simulink model "bwb11"  (Simulink 7.8)
settings: Solver=ode45  StartTime=0.0  StopTime=10.0  RelTol=1e-3
values from neighbouring files (symbols this model uses):
  eagleray = aerosonde_data    [aerosonde_initialize.m]
  euler_0 = [theta_trim; 0; 0]    [aerosonde_initialize.m]
  fuel_0 = 2    [aerosonde_initialize.m]
  Omega_0 = 5000*pi/30    (= 523.598775598)    [aerosonde_initialize.m]
  position_0 = [0; 0; -h_trim]    [aerosonde_initialize.m]
  rates_0 = [0; q_trim ; 0]    [aerosonde_initialize.m]
  velocity_0 = [23; 0; 0]    [aerosonde_initialize.m]
undefined symbols (not defined in the file or in its folder): ke, rAC, tc, z
libraries: aerolibasang x3, aerolibadynsys x3, aerolibbdyn x2, aerolibutil x2, aerolibtransform2 x1, aerolib6dof2 x1, aerolibatmos2 x1
settings Model: Creator=Shihan Tissera  LastModifiedBy=s153429
settings OptimizationCC: InitFltsAndDblsToZero=on
settings DebuggingCC: FcnCallInpInsideContextMsg=Use local settings  StrictBusMsg=Warning

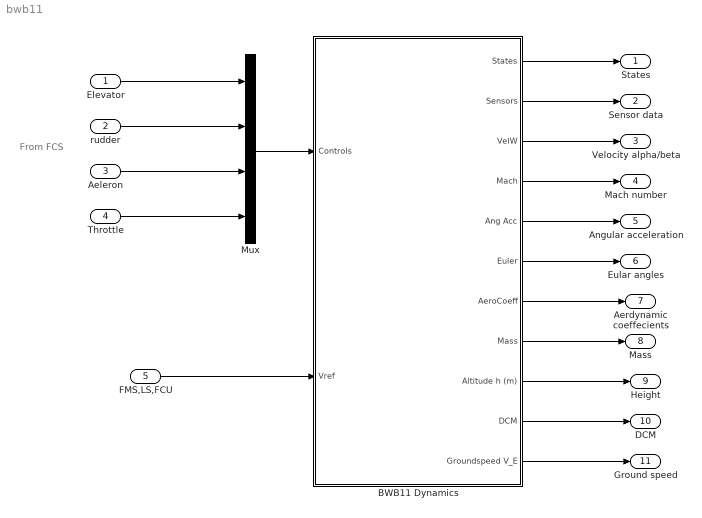
== system bwb11 ==
  note: From FCS
  Elevator : Inport
  rudder : Inport  Port=2
  Aeleron : Inport  Port=3
  Throttle : Inport  Port=4
  FMS,LS,FCU : Inport  Port=5
  BWB11 Dynamics : Subsystem  mask(6-DOF Aerosonde Model){as=eagleray, Velocities0=velocity_0, Rates0=rates_0, Euler0=euler_0, Position0=position_0, Fuel0=fuel_0, Omega0=Omega_0, GndAlt=0}
      mask prompts: as "Aircraft configuration data:"; Velocities0 "Initial velocity in body axes [u,v,w]: (m/s)"; Rates0 "Initial body rotation rates [p,q,r]: (rad/s)"; Euler0 "Initial Euler orientation [roll, pitch, yaw]: (rad)"; Position0 "Initial position in inertial axes [Xe,Ye,Ze]: (m)"; Fuel0 "Initial fuel mass: (Kg)"; Omega0 "Initial engine speed: (rad/s)"; GndAlt "Ground altitude: (m)"
      mask help:
      | Nonlinear 6-DOF Aerosonde  model with equations of motion in
      | body frame.
      |
      | Version 2011a (18 February 2011)
      mask Help:
      | The block implements the 6-DOF nonlinear Aerosonde model. It is an adaptation of the model provided in the AeroSim blockset. Velocities are computed in body frame.
      | <P><B>Inputs:</B>
      | <LI>Controls = the 4x1 vector of aircraft controls [elevator aileron rudder throttle]. Aerodynamic controls are in radians, throttle is from 0 to 1.</LI>
      | <LI>RST = the integrator reset flag (0 or 1, all integrators on rising edge)
      | <LI>V_wind = the 3x1 vector of background wind speed components in navigation frame [North East Down]</LI>
      | <LI>omega_wind = the 3x1 vector of background wind angular rates in navigation frame [North East Down]</LI>
      | </P>
      | <P><B>Outputs:</B>
      | <LI>States = the 14x1 aircraft state vector [Velocities, Angular rates, Euler angles, Position, Fuel mass, Engine speed].</LI>
      | <LI>Sensors = the 15x1 vector of sensor outputs [GPS Position, GPS Groundspeed, Accelerometers, Gyros, Air data].</LI>
      | <LI>VelW = the 3x1 vector of aircraft velocity in wind axes [Airspeed, sideslip, angle of attack]</LI>
      | <LI>Mach = the Mach number</LI>
      | <LI>Ang Acc = the 3x1 vector of angular accelerations
      | <LI>Euler = the 3x1 vector of Euler angles (roll, pitch, yaw)</LI>
      | <LI>AeroCoeff = the 6x1 vector of aerodynamic coefficients [CD CY CL Cl Cm Cn]</LI>
      | <LI>Mass = the current aircraft mass</LI>
      | <LI>h = the aircraft altitude</LI>
      | </P>
      | <P><B>Parameters:</B>
      | <LI>Aircraft configuration data = structured varaible with aircraft data<BR>
      | obtain by  ``aerosonde=aerosonde_initialize'' for example</LI>
      | <LI>Initial velocities = the 3x1 vector of initial aircraft velocities in body axes [u v w]</LI>
      | <LI>Initial angular rates = the 3x1 vector of initial angular rates [p q r]</LI>
      | <LI>Initial attitude = the 3x1 vector of initial Euler angles [phi theta psi]</LI>
      | <LI>Initial position = the 3x1 vector of initial aircraft location [Lat Lon Alt]</LI>
      | <LI>Initial fuel mass = the initial quantity of fuel on-board the aircraft</LI>
      | <LI>Initial engine speed = the initial engine rotation speed</LI>
      | <LI>Ground altitude = the ground altitude at aircraft location</LI>
      | </P>
      | <P>
      | <I>Version 2010b (26 May 2010)</I>
      | </P>
  Mux : Mux
  States : Outport
  Sensor data : Outport  Port=2
  Velocity alpha/beta : Outport  Port=3
  Mach number : Outport  Port=4
  Angular acceleration : Outport  Port=5
  Eular angles : Outport  Port=6
  Aerdynamic coeffecients : Outport  Port=7
  Mass : Outport  Port=8
  Height : Outport  Port=9
  DCM : Outport  Port=10
  Ground speed : Outport  Port=11
  wires:
  BWB11 Dynamics/1(States) -> States/1
  BWB11 Dynamics/2(Sensors) -> Sensor data/1
  BWB11 Dynamics/3(VelW) -> Velocity alpha/beta/1
  BWB11 Dynamics/4(Mach) -> Mach number/1
  BWB11 Dynamics/5(Ang Acc) -> Angular acceleration/1
  BWB11 Dynamics/6(Euler) -> Eular angles/1
  BWB11 Dynamics/7(AeroCoeff) -> Aerdynamic coeffecients/1
  BWB11 Dynamics/8(Mass) -> Mass/1
  BWB11 Dynamics/9("Altitude h (m) ") -> Height/1
  BWB11 Dynamics/10(DCM) -> DCM/1
  BWB11 Dynamics/11(Groundspeed V_E) -> Ground speed/1
  Mux/1 -> BWB11 Dynamics/1(Controls)
  Elevator/1 -> Mux/1
  rudder/1 -> Mux/2
  Aeleron/1 -> Mux/3
  Throttle/1 -> Mux/4
  FMS,LS,FCU/1 -> BWB11 Dynamics/2(Vref)

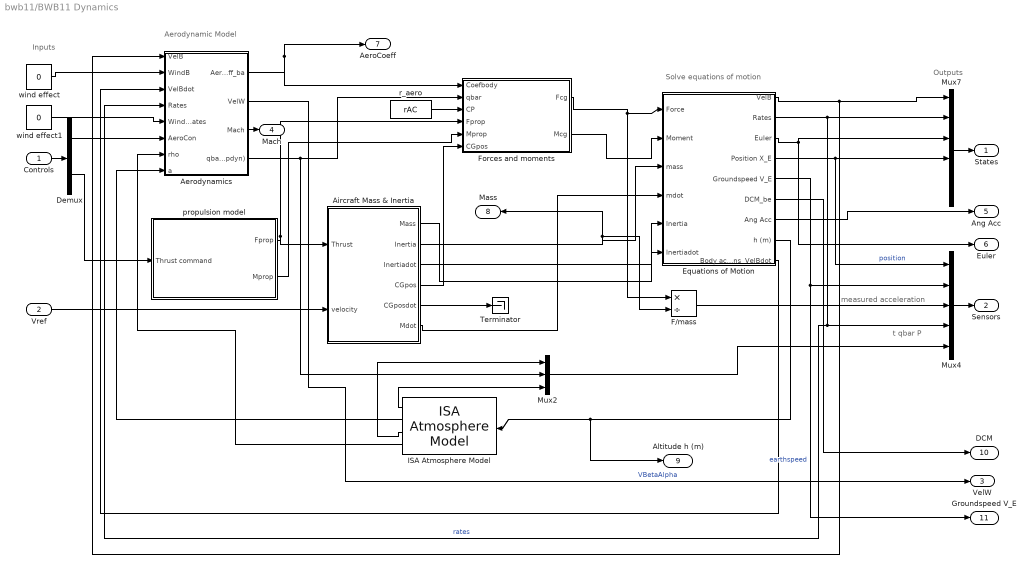
== system bwb11/BWB11 Dynamics ==
  note: t qbar P
  note: measured acceleration
  note: Aerodynamic Model
  note: Outputs
  note: Inputs
  note: Solve equations of motion
  Controls : Inport
  Vref : Inport  Port=2
  Aerodynamics : Subsystem
  Aircraft Mass & Inertia : Subsystem
  Demux : Demux  Outputs=[4,3]
  Equations of Motion : Subsystem
  F/mass : Product  Inputs=*/  RndMeth=Zero
  Forces and moments : Subsystem
  ISA Atmosphere Model : aerolibatmos2/ISA Atmosphere Model  custom=off  g=9.80665  gamma=1.4  R=287.0531  L=0.0065  h_trop=11000  h_strat=20000  rho0=1.225  P0=101325  T0=288.15
  Mux2 : Mux  Inputs=3
  Mux4 : Mux  Inputs=5
  Mux7 : Mux  Inputs=6
  Terminator : Terminator
  propulsion model : Subsystem
  r_aero : Constant  Value=rAC
  wind effect : Constant  Value=0
  wind effect1 : Constant  Value=0
  States : Outport
  Sensors : Outport  Port=2
  VelW : Outport  Port=3
  Mach : Outport  Port=4
  Ang Acc : Outport  Port=5
  Euler : Outport  Port=6
  AeroCoeff : Outport  Port=7
  Mass : Outport  Port=8
  "Altitude h (m) " : Outport  Port=9
  DCM : Outport  Port=10
  Groundspeed V_E : Outport  Port=11
  wires:
  wind effect/1 -> Aerodynamics/2(WindB)
  wind effect1/1 -> Aerodynamics/5(WindRates)
  Equations of Motion/9(Body accns  VelBdot) -> Aerodynamics/3(VelBdot)
  F/mass/1 -> Mux4/3
  Aircraft Mass & Inertia/2(Inertia) -> Equations of Motion/5(Inertia)
  Forces and moments/1(Fcg) -> F/mass/1, Equations of Motion/1(Force)
  r_aero/1 -> Forces and moments/3(CP)
  Equations of Motion/8(h (m)) -> "Altitude h (m) "/1, ISA Atmosphere Model/1
  ISA Atmosphere Model/4 -> Aerodynamics/7(rho)
  ISA Atmosphere Model/3 -> Mux2/1
  ISA Atmosphere Model/2 -> Aerodynamics/8("a ")
  ISA Atmosphere Model/1 -> Mux2/3
  Aerodynamics/1(AeroCoeff_ba) -> AeroCoeff/1, Forces and moments/1(Coefbody)
  Aerodynamics/3(Mach) -> Mach/1
  Demux/1 -> Aerodynamics/6(AeroCon)
  Equations of Motion/4(Position X_E) -> Mux4/1, Mux7/4  "position"
  Equations of Motion/2(Rates) -> Mux7/2, Mux4/4, Aerodynamics/4(Rates)  "rates"
  Equations of Motion/1(VelB) -> Aerodynamics/1(VelB), Mux7/1
  Demux/2 -> propulsion model/1(Thrust command)
  Mux7/1 -> States/1
  Mux4/1 -> Sensors/1
  Controls/1 -> Demux/1
  Equations of Motion/5(Groundspeed V_E) -> Groundspeed V_E/1, Mux4/2  "earthspeed"
  Aircraft Mass & Inertia/1(Mass) -> F/mass/2, Equations of Motion/3(mass), Mass/1
  Forces and moments/2(Mcg) -> Equations of Motion/2(Moment)
  propulsion model/1(Fprop) -> Forces and moments/4(Fprop), Aircraft Mass & Inertia/1(Thrust)
  propulsion model/2(Mprop) -> Forces and moments/5(Mprop)
  Equations of Motion/6(DCM_be) -> DCM/1
  Aerodynamics/4(qbar (pdyn)) -> Mux2/2, Forces and moments/2(qbar)
  Mux2/1 -> Mux4/5
  Aerodynamics/2(VelW) -> VelW/1  "VBetaAlpha"
  Equations of Motion/7(Ang Acc) -> Ang Acc/1
  Equations of Motion/3(Euler) -> Mux7/3, Euler/1
  Aircraft Mass & Inertia/4(CGpos) -> Forces and moments/6(CGpos)
  Aircraft Mass & Inertia/6(Mdot) -> Equations of Motion/4(mdot)
  Aircraft Mass & Inertia/5(CGposdot) -> Terminator/1
  Aircraft Mass & Inertia/3(Inertiadot) -> Equations of Motion/6(Inertiadot)
  Vref/1 -> Aircraft Mass & Inertia/2(velocity)

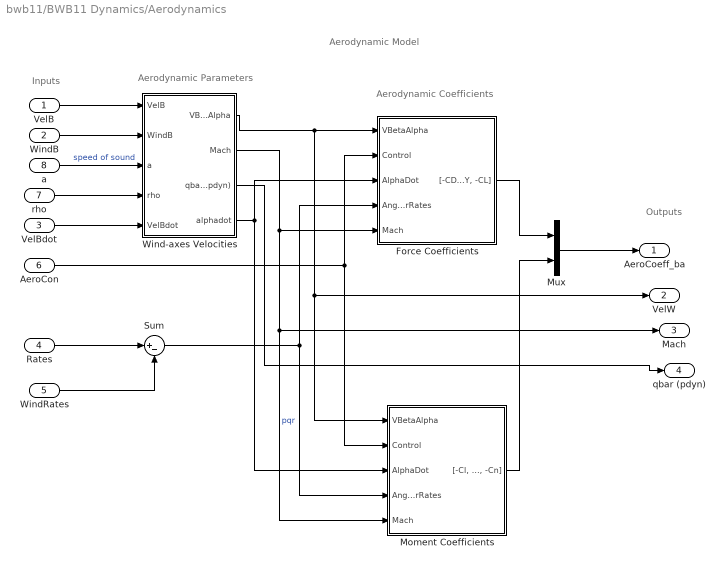
== system bwb11/BWB11 Dynamics/Aerodynamics ==
  note: Aerodynamic Model
  note: Aerodynamic Coefficients
  note: Aerodynamic Parameters
  note: Outputs
  note: Inputs
  VelB : Inport  PortDimensions=[3 1]
  WindB : Inport  Port=2  PortDimensions=[3 1]
  VelBdot : Inport  Port=3
  Rates : Inport  Port=4  PortDimensions=[3 1]
  WindRates : Inport  Port=5  PortDimensions=[3 1]
  AeroCon : Inport  Port=6  PortDimensions=[4 1]
  rho : Inport  Port=7  PortDimensions=1
  "a " : Inport  Port=8  PortDimensions=1
  Force Coefficients : Subsystem
  Moment Coefficients : Subsystem
  Mux : Mux  Inputs=2
  Sum : Sum  Inputs=|+-  SaturateOnIntegerOverflow=on  InputSameDT=on  OutDataTypeStr=Inherit: Same as first input
  Wind-axes Velocities : Subsystem
  AeroCoeff_ba : Outport
  VelW : Outport  Port=2
  Mach : Outport  Port=3
  qbar (pdyn) : Outport  Port=4
  wires:
  VelBdot/1 -> Wind-axes Velocities/5(VelBdot)
  Wind-axes Velocities/4(alphadot) -> Force Coefficients/3(AlphaDot), Moment Coefficients/3(AlphaDot)
  WindB/1 -> Wind-axes Velocities/2(WindB)
  Mux/1 -> AeroCoeff_ba/1
  Moment Coefficients/1("[-Cl, Cm, -Cn]") -> Mux/2
  Force Coefficients/1("[-CD, CY, -CL]") -> Mux/1
  rho/1 -> Wind-axes Velocities/4(rho)
  VelB/1 -> Wind-axes Velocities/1(VelB)
  "a "/1 -> Wind-axes Velocities/3(a)  "speed of sound"
  Wind-axes Velocities/1(VBetaAlpha) -> Moment Coefficients/1(VBetaAlpha), VelW/1, Force Coefficients/1(VBetaAlpha)
  AeroCon/1 -> Moment Coefficients/2(Control), Force Coefficients/2(Control)
  Wind-axes Velocities/2(Mach) -> Moment Coefficients/5(Mach), Force Coefficients/5(Mach), Mach/1
  Wind-axes Velocities/3(qbar (pdyn)) -> qbar (pdyn)/1
  Rates/1 -> Sum/1
  Sum/1 -> Moment Coefficients/4(AngularRates), Force Coefficients/4(AngularRates)  "pqr"
  WindRates/1 -> Sum/2

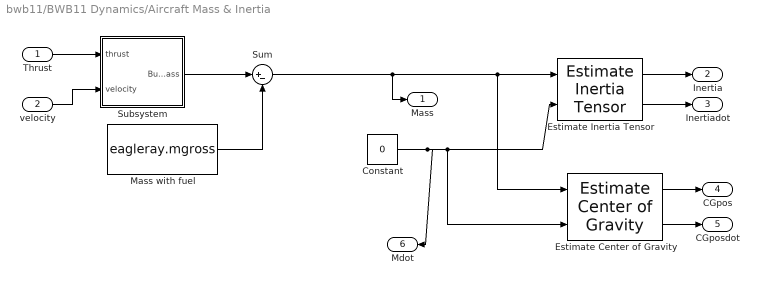
== system bwb11/BWB11 Dynamics/Aircraft Mass & Inertia ==
  Thrust : Inport
  velocity : Inport  Port=2
  Constant : Constant  Value=0
  Estimate Center of Gravity : aerolibbdyn/Estimate Center of Gravity  fmass=eagleray.mgross  emass=eagleray.mempty  fcg=eagleray.CGgross  ecg=eagleray.CGempty
  Estimate Inertia Tensor : aerolibbdyn/Estimate Inertia Tensor  fmass=eagleray.mgross  emass=eagleray.mempty  fI=eagleray.Jgross  eI=eagleray.Jempty
  Mass with fuel : Constant  Value=eagleray.mgross
  Subsystem : Subsystem
  Sum : Sum  Inputs=|+-  SaturateOnIntegerOverflow=on  InputSameDT=on  OutDataTypeStr=Inherit: Same as first input
  Mass : Outport
  Inertia : Outport  Port=2
  Inertiadot : Outport  Port=3
  CGpos : Outport  Port=4
  CGposdot : Outport  Port=5
  Mdot : Outport  Port=6
  wires:
  Estimate Center of Gravity/2 -> CGposdot/1
  Estimate Center of Gravity/1 -> CGpos/1
  Estimate Inertia Tensor/2 -> Inertiadot/1
  Estimate Inertia Tensor/1 -> Inertia/1
  Sum/1 -> Estimate Center of Gravity/1, Estimate Inertia Tensor/1, Mass/1
  Mass with fuel/1 -> Sum/2
  Subsystem/1(Burned fuel mass) -> Sum/1
  Constant/1 -> Estimate Inertia Tensor/2, Estimate Center of Gravity/2, Mdot/1
  Thrust/1 -> Subsystem/1(thrust)
  velocity/1 -> Subsystem/2(velocity)

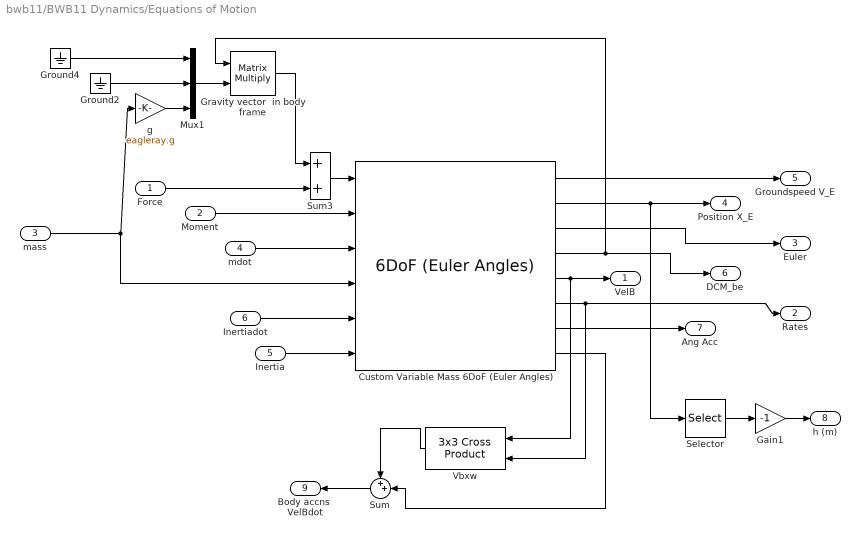
== system bwb11/BWB11 Dynamics/Equations of Motion ==
  Force : Inport  PortDimensions=3
  Moment : Inport  Port=2  PortDimensions=3
  mass : Inport  Port=3  PortDimensions=1
  mdot : Inport  Port=4  PortDimensions=1
  Inertia : Inport  Port=5  PortDimensions=[3,3]
  Inertiadot : Inport  Port=6  PortDimensions=[3,3]
  Custom Variable Mass 6DoF (Euler Angles) : aerolib6dof2/6DoF (Euler Angles)  units=Metric (MKS)  mtype=Custom Variable  rep=Euler Angles  xme_0=Position0  Vm_0=Velocities0  eul_0=Euler0  pm_0=Rates0  mass_0=1.0  mass_e=0  mass_f=0  inertia=eye(3)  inertia_e=eye(3)  inertia_f=eye(3)  k_quat=1.0
  Gain1 : Gain  Gain=-1
  "Gravity vector  in body frame " : Product  Multiplication=Matrix(*)  SaturateOnIntegerOverflow=on  InputSameDT=on  OutDataTypeStr=Inherit: Same as first input
  Ground2 : Ground
  Ground4 : Ground
  Mux1 : Mux  Inputs=3
  Selector : Selector  InputPortWidth=3  IndexOptions=Index vector (dialog)  Indices=3  OutputSizes=1
  Sum : Sum  Inputs=++|  SaturateOnIntegerOverflow=on
  Sum3 : Sum  SaturateOnIntegerOverflow=on  InputSameDT=on  OutDataTypeStr=Inherit: Same as first input
  Vbxw : aerolibutil/3x3 Cross Product
  g : Gain  Gain=eagleray.g
  VelB : Outport
  Rates : Outport  Port=2
  Euler : Outport  Port=3
  Position X_E : Outport  Port=4
  Groundspeed V_E : Outport  Port=5
  DCM_be : Outport  Port=6
  Ang Acc : Outport  Port=7
  h (m) : Outport  Port=8
  Body accns  VelBdot : Outport  Port=9
  wires:
  Vbxw/1 -> Sum/1
  Sum/1 -> Body accns  VelBdot/1
  Custom Variable Mass 6DoF (Euler Angles)/8 -> Sum/2
  Custom Variable Mass 6DoF (Euler Angles)/7 -> Ang Acc/1
  Custom Variable Mass 6DoF (Euler Angles)/6 -> Vbxw/2, Rates/1
  Inertia/1 -> Custom Variable Mass 6DoF (Euler Angles)/6
  mdot/1 -> Custom Variable Mass 6DoF (Euler Angles)/3
  Gain1/1 -> h (m)/1
  Selector/1 -> Gain1/1
  Sum3/1 -> Custom Variable Mass 6DoF (Euler Angles)/1
  g/1 -> Mux1/3
  "Gravity vector  in body frame "/1 -> Sum3/1
  Custom Variable Mass 6DoF (Euler Angles)/3 -> Euler/1
  Custom Variable Mass 6DoF (Euler Angles)/2 -> Selector/1, Position X_E/1
  Custom Variable Mass 6DoF (Euler Angles)/1 -> Groundspeed V_E/1
  Custom Variable Mass 6DoF (Euler Angles)/5 -> Vbxw/1, VelB/1
  Ground4/1 -> Mux1/1
  Ground2/1 -> Mux1/2
  mass/1 -> Custom Variable Mass 6DoF (Euler Angles)/4, g/1
  Custom Variable Mass 6DoF (Euler Angles)/4 -> DCM_be/1, "Gravity vector  in body frame "/1
  Mux1/1 -> "Gravity vector  in body frame "/2
  Force/1 -> Sum3/2
  Moment/1 -> Custom Variable Mass 6DoF (Euler Angles)/2
  Inertiadot/1 -> Custom Variable Mass 6DoF (Euler Angles)/5

== system bwb11/BWB11 Dynamics/Forces and moments ==
  Coefbody : Inport
  qbar : Inport  Port=2
  CP : Inport  Port=3
  Fprop : Inport  Port=4
  Mprop : Inport  Port=5
  CGpos : Inport  Port=6
  Aerodynamic Forces and Moments : Subsystem  AncestorBlock=aerolibadyn/Aerodynamic Forces and Moments  mask(Aerodynamic Forces and Moments){inputAxes=Body, outputForceAxes=Body, outputMomentAxes=Body, S=eagleray.S, b=eagleray.b, cbar=eagleray.MAC}
      mask prompts: inputAxes "Input axes:"; outputForceAxes "Force axes:"; outputMomentAxes "Moment axes:"; S "Reference area:"; b "Reference span:"; cbar "Reference length:"
      mask help: Compute the aerodynamic forces and moments applied at the center of gravity using the aerodynamic coefficients, dynamic pressure, center of gravity and center of pressure.
      mask init:
      | ports=aeroicon('aeroblkadyn','icon');
      mask Help: eval('asbhelp');
      mask StyleString: popup(Body|Stability|Wind),popup(Body|Stability|Wind),popup(Body|Stability|Wind),edit,edit,edit
      mask Display:
      | port_label(ports(1).type,ports(1).port,ports(1).txt,'texmode','on');
      | port_label(ports(2).type,ports(2).port,ports(2).txt,'texmode','on');
      | port_label(ports(3).type,ports(3).port,ports(3).txt,'texmode','on');
      | port_label(ports(4).type,ports(4).port,ports(4).txt,'texmode','on');
      | port_label(ports(5).type,ports(5).port,ports(5).txt,'texmode','on');
      | port_label(ports(6).type,ports(6).port,ports(6).txt,'texmode','on');
      | port_label(ports(7).type,ports(7).port,ports(7).txt,'texmode','on');
  Total Moment : Subsystem
  Fcg : Outport
  Mcg : Outport  Port=2
  wires:
  Aerodynamic Forces and Moments/2(Moments) -> Total Moment/2(Maero)
  Aerodynamic Forces and Moments/1(Forces) -> Total Moment/1(Faero)
  CGpos/1 -> Total Moment/5(CGpos), Aerodynamic Forces and Moments/3(CG)
  Coefbody/1 -> Aerodynamic Forces and Moments/1(Coefficients)
  qbar/1 -> Aerodynamic Forces and Moments/2(qbar)
  CP/1 -> Aerodynamic Forces and Moments/4(CP)
  Fprop/1 -> Total Moment/3(Fprop)
  Mprop/1 -> Total Moment/4(Mprop)
  Total Moment/2(Mcg) -> Mcg/1
  Total Moment/1(Fcg) -> Fcg/1

== system bwb11/BWB11 Dynamics/propulsion model ==
  Thrust command : Inport
  CGtoFdistance : Constant  Value=z
  Engine model : TransferFcn  Numerator=[ke]  Denominator=[tc 1]
  Product : Product  RndMeth=Zero
  Fprop : Outport
  Mprop : Outport  Port=2
  wires:
  CGtoFdistance/1 -> Product/2
  Engine model/1 -> Product/1, Fprop/1
  Product/1 -> Mprop/1
  Thrust command/1 -> Engine model/1

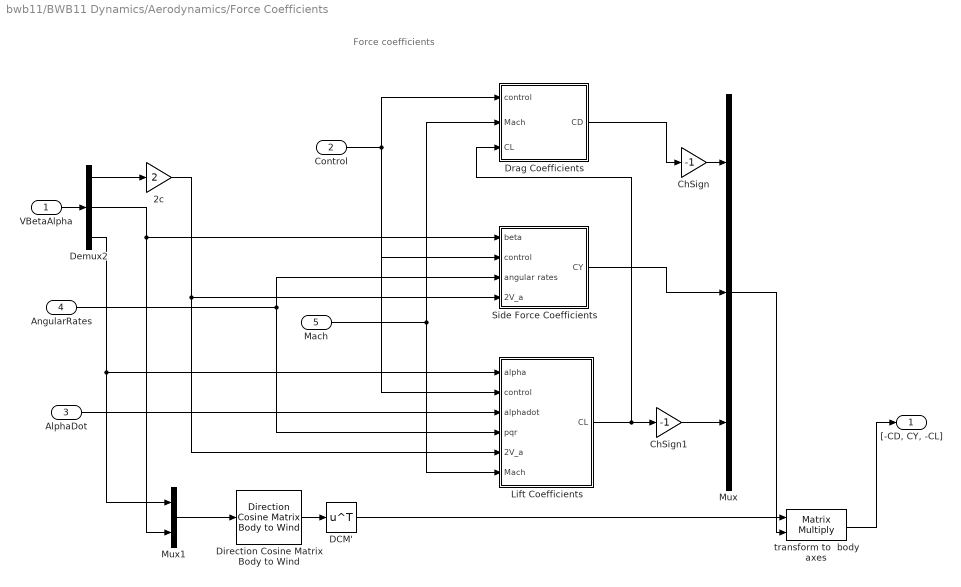
== system bwb11/BWB11 Dynamics/Aerodynamics/Force Coefficients ==
  note: Force coefficients
  VBetaAlpha : Inport  PortDimensions=[3 1]
  Control : Inport  Port=2  PortDimensions=[4 1]
  AlphaDot : Inport  Port=3
  AngularRates : Inport  Port=4  PortDimensions=[3 1]
  Mach : Inport  Port=5  PortDimensions=1
  2c : Gain  Gain=2  SaturateOnIntegerOverflow=on  OutDataTypeStr=Inherit: Same as input  ParamDataTypeStr=Inherit: Same as input
  ChSign : Gain  Gain=-1  SaturateOnIntegerOverflow=on  OutDataTypeStr=Inherit: Same as input  ParamDataTypeStr=Inherit: Same as input
  ChSign1 : Gain  Gain=-1  SaturateOnIntegerOverflow=on  OutDataTypeStr=Inherit: Same as input  ParamDataTypeStr=Inherit: Same as input
  DCM' : Math  Operator=transpose  SaturateOnIntegerOverflow=on
  Demux2 : Demux  Outputs=3
  Direction Cosine Matrix Body to Wind : aerolibtransform2/Direction Cosine Matrix Body to Wind
  Drag Coefficients : Subsystem
  Lift Coefficients : Subsystem
  Mux : Mux  Inputs=3
  Mux1 : Mux  Inputs=2
  Side Force Coefficients : Subsystem
  transform to  body axes : Product  Inputs=**  Multiplication=Matrix(*)  SaturateOnIntegerOverflow=on  InputSameDT=on  OutDataTypeStr=Inherit: Same as first input
  "[-CD, CY, -CL]" : Outport
  wires:
  Mux1/1 -> Direction Cosine Matrix Body to Wind/1
  DCM'/1 -> transform to  body axes/1
  Mux/1 -> transform to  body axes/2
  Direction Cosine Matrix Body to Wind/1 -> DCM'/1
  transform to  body axes/1 -> "[-CD, CY, -CL]"/1
  Demux2/2 -> Mux1/2, Side Force Coefficients/1(beta)
  Demux2/1 -> 2c/1
  VBetaAlpha/1 -> Demux2/1
  ChSign1/1 -> Mux/3
  ChSign/1 -> Mux/1
  Side Force Coefficients/1(CY) -> Mux/2
  Drag Coefficients/1(CD) -> ChSign/1
  Lift Coefficients/1(CL) -> Drag Coefficients/3(CL), ChSign1/1
  Mach/1 -> Drag Coefficients/2(Mach), Lift Coefficients/6(Mach)
  AngularRates/1 -> Side Force Coefficients/3(angular rates), Lift Coefficients/4(pqr)
  AlphaDot/1 -> Lift Coefficients/3(alphadot)
  Control/1 -> Lift Coefficients/2(control), Side Force Coefficients/2(control), Drag Coefficients/1(control)
  Demux2/3 -> Lift Coefficients/1(alpha), Mux1/1
  2c/1 -> Side Force Coefficients/4(2V_a), Lift Coefficients/5(2V_a)

== system bwb11/BWB11 Dynamics/Aerodynamics/Moment Coefficients ==
  note: Moment coefficients
  VBetaAlpha : Inport  PortDimensions=[3 1]
  Control : Inport  Port=2  PortDimensions=[4 1]
  AlphaDot : Inport  Port=3
  AngularRates : Inport  Port=4  PortDimensions=[3 1]
  Mach : Inport  Port=5  PortDimensions=1
  2c : Gain  Gain=2  SaturateOnIntegerOverflow=on  OutDataTypeStr=Inherit: Same as input  ParamDataTypeStr=Inherit: Same as input
  Demux1 : Demux  Outputs=3
  Mux : Mux  Inputs=3
  Pitch Moment Coefficients : Subsystem
  Roll Moment Coefficients : Subsystem
  Yaw Moment Coefficients : Subsystem
  "[-Cl, Cm, -Cn]" : Outport
  wires:
  Demux1/2 -> Yaw Moment Coefficients/1(beta), Roll Moment Coefficients/1(beta)
  Demux1/3 -> Pitch Moment Coefficients/1(alpha)
  Mach/1 -> Pitch Moment Coefficients/6(Mach)
  Yaw Moment Coefficients/1(Cn) -> Mux/3
  VBetaAlpha/1 -> Demux1/1
  2c/1 -> Pitch Moment Coefficients/5(2V_a), Yaw Moment Coefficients/4(2V_a), Roll Moment Coefficients/4(2V)
  Demux1/1 -> 2c/1
  Control/1 -> Roll Moment Coefficients/2(control), Yaw Moment Coefficients/2(control), Pitch Moment Coefficients/2(control)
  AlphaDot/1 -> Pitch Moment Coefficients/3(alphadot)
  AngularRates/1 -> Roll Moment Coefficients/3(angular rates), Yaw Moment Coefficients/3(angular rates), Pitch Moment Coefficients/4(pqr)
  Mux/1 -> "[-Cl, Cm, -Cn]"/1
  Pitch Moment Coefficients/1(Cm) -> Mux/2
  Roll Moment Coefficients/1(Cl) -> Mux/1

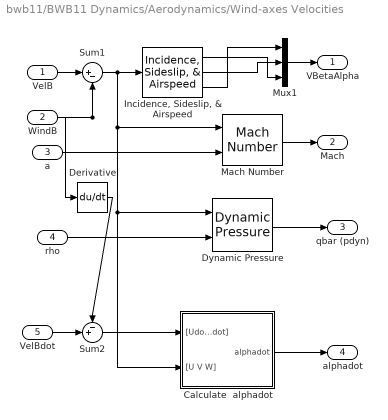
== system bwb11/BWB11 Dynamics/Aerodynamics/Wind-axes Velocities ==
  VelB : Inport
  WindB : Inport  Port=2
  a : Inport  Port=3
  rho : Inport  Port=4
  VelBdot : Inport  Port=5
  Calculate  alphadot : Subsystem
  Derivative : Derivative
  Dynamic Pressure : aerolibasang/Dynamic Pressure
  "Incidence, Sideslip, & Airspeed" : aerolibasang/Incidence, Sideslip, & Airspeed
  Mach Number : aerolibasang/Mach Number
  Mux1 : Mux  Inputs=3
  Sum1 : Sum  Inputs=|+-  SaturateOnIntegerOverflow=on  InputSameDT=on  OutDataTypeStr=Inherit: Same as first input
  Sum2 : Sum  Inputs=-+|  SaturateOnIntegerOverflow=on  InputSameDT=on  OutDataTypeStr=Inherit: Same as first input
  VBetaAlpha : Outport
  Mach : Outport  Port=2
  qbar (pdyn) : Outport  Port=3
  alphadot : Outport  Port=4
  wires:
  Derivative/1 -> Sum2/1
  Sum2/1 -> Calculate  alphadot/1("[Udot Vdot Wdot]")
  VelBdot/1 -> Sum2/2
  Calculate  alphadot/1(alphadot) -> alphadot/1
  "Incidence, Sideslip, & Airspeed"/2 -> Mux1/2
  "Incidence, Sideslip, & Airspeed"/1 -> Mux1/3
  Dynamic Pressure/1 -> qbar (pdyn)/1
  rho/1 -> Dynamic Pressure/2
  a/1 -> Mach Number/2
  Mach Number/1 -> Mach/1
  WindB/1 -> Derivative/1, Sum1/2
  VelB/1 -> Sum1/1
  Mux1/1 -> VBetaAlpha/1
  "Incidence, Sideslip, & Airspeed"/3 -> Mux1/1
  Sum1/1 -> Calculate  alphadot/2("[U V W]"), Dynamic Pressure/1, Mach Number/1, "Incidence, Sideslip, & Airspeed"/1

== system bwb11/BWB11 Dynamics/Aircraft Mass & Inertia/Subsystem ==
  thrust : Inport
  velocity : Inport  Port=2
  Divide : Product  Inputs=*/
  Integrator : Integrator
  Product : Product  RndMeth=Zero
  Product1 : Product  RndMeth=Zero
  calerific value : Constant  Value=eagleray.cali
  "efficency " : Constant  Value=eagleray.Efi
  Burned fuel mass : Outport
  wires:
  thrust/1 -> Product/1
  velocity/1 -> Product/2
  Product/1 -> Integrator/1
  Integrator/1 -> Product1/1
  Divide/1 -> Product1/2
  Product1/1 -> Burned fuel mass/1
  "efficency "/1 -> Divide/1
  calerific value/1 -> Divide/2

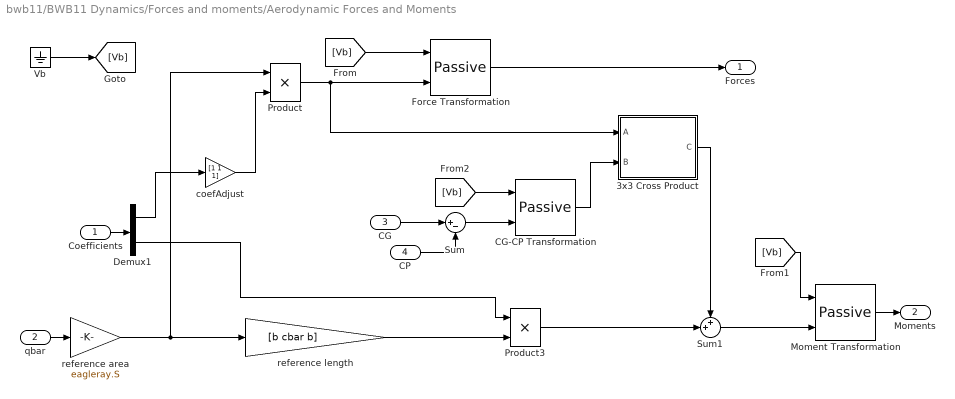
== system bwb11/BWB11 Dynamics/Forces and moments/Aerodynamic Forces and Moments ==
  Coefficients : Inport
  qbar : Inport  Port=2
  CG : Inport  Port=3
  CP : Inport  Port=4
  3x3 Cross Product : Subsystem  AncestorBlock=aerolibutil/3x3 Cross Product  mask(CrossProduct){}
      mask help: Calculate the cross product of two 3-by-1 vectors.
      mask init:
      | aeroicon('aeroblk');
      mask Help: eval('asbhelp(''threebythree_cross_product'')');
      mask Display:
      | text(.5,.5,'Cross\nProduct\nC = AxB', ...
      | 	'HorizontalAlignment','Center',...
      | 	'VerticalAlignment','middle')
  CG-CP Transformation : aerolibadynsys/Passive  SystemSampleTime=-1
  Demux1 : Demux  Outputs=[3,3]
  Force Transformation : aerolibadynsys/Passive  SystemSampleTime=-1
  Moment Transformation : aerolibadynsys/Passive  SystemSampleTime=-1
  Product : Product  SaturateOnIntegerOverflow=on  InputSameDT=on  OutDataTypeStr=Inherit: Same as first input
  Product3 : Product  SaturateOnIntegerOverflow=on  InputSameDT=on  OutDataTypeStr=Inherit: Same as first input
  Sum : Sum  Inputs=|+-  SaturateOnIntegerOverflow=on
  Sum1 : Sum  Inputs=++|  SaturateOnIntegerOverflow=on  InputSameDT=on  OutDataTypeStr=Inherit: Same as first input
  Vb : Ground
  coefAdjust : Gain  Gain="[1  1  1]"
  reference area : Gain  Gain=eagleray.S  SaturateOnIntegerOverflow=on  OutDataTypeStr=Inherit: Same as input  ParamDataTypeStr=Inherit: Same as input
  reference length : Gain  Gain=[b cbar b]  SaturateOnIntegerOverflow=on  OutDataTypeStr=Inherit: Same as input  ParamDataTypeStr=Inherit: Same as input
  Forces : Outport
  Moments : Outport  Port=2
  wires:
  3x3 Cross Product/1(C) -> Sum1/1
  reference length/1 -> Product3/2
  Coefficients/1 -> Demux1/1
  Demux1/2 -> Product3/1
  qbar/1 -> reference area/1
  reference area/1 -> reference length/1, Product/1
  Product3/1 -> Sum1/2
  Demux1/1 -> coefAdjust/1
  Product/1 -> Force Transformation/2, 3x3 Cross Product/1(A)
  Force Transformation/1 -> Forces/1
  Vb/1 -> [Vb]
  [Vb] -> Force Transformation/1
  Sum1/1 -> Moment Transformation/2
  Moment Transformation/1 -> Moments/1
  [Vb] -> Moment Transformation/1
  coefAdjust/1 -> Product/2
  CG/1 -> Sum/1
  CP/1 -> Sum/2
  Sum/1 -> CG-CP Transformation/2
  CG-CP Transformation/1 -> 3x3 Cross Product/2(B)
  [Vb] -> CG-CP Transformation/1

== system bwb11/BWB11 Dynamics/Forces and moments/Total Moment ==
  note: Sum forces and moments
  note: Total moments at CG location
  Faero : Inport  PortDimensions=3
  Maero : Inport  Port=2  PortDimensions=3
  Fprop : Inport  Port=3  PortDimensions=3
  Mprop : Inport  Port=4  PortDimensions=3
  CGpos : Inport  Port=5  PortDimensions=3
  Moments about CG  due to Propulsion   Forces : Subsystem  AncestorBlock="aerolibbdyn/Moments about CG  due to Forces"  mask(Moments About CG Due To Forces){}
      mask help: Compute moments about center of gravity due to forces which are applied at point CP not the center of gravity.
      mask init:
      | [xpw ypw xp yp x y]=aeroimage('momcg');
      mask Help: web(asbhelp);
      mask Display:
      | port_label('input',1,'F','texmode','on');
      | port_label('input',2,'CG','texmode','on');
      | port_label('input',3,'CP','texmode','on');
      | port_label('output',1,'M','texmode','on');
      | patch(xp,yp);
      | patch(xpw,ypw,[1 1 1]);
      | plot(x,y);
  Sum1 : Sum  Inputs=+++  SaturateOnIntegerOverflow=on  InputSameDT=on  OutDataTypeStr=Inherit: Same as first input
  Total forces  (excluding g) : Sum  SaturateOnIntegerOverflow=on  InputSameDT=on  OutDataTypeStr=Inherit: Same as first input
  Fcg : Outport
  Mcg : Outport  Port=2
  wires:
  Maero/1 -> Sum1/2
  Moments about CG  due to Propulsion   Forces/1(Moments) -> Sum1/1
  Total forces  (excluding g)/1 -> Fcg/1
  Faero/1 -> Total forces  (excluding g)/1
  Fprop/1 -> Total forces  (excluding g)/2, Moments about CG  due to Propulsion   Forces/1(Forces)
  Mprop/1 -> Sum1/3
  Sum1/1 -> Mcg/1
  CGpos/1 -> Moments about CG  due to Propulsion   Forces/2(CG)

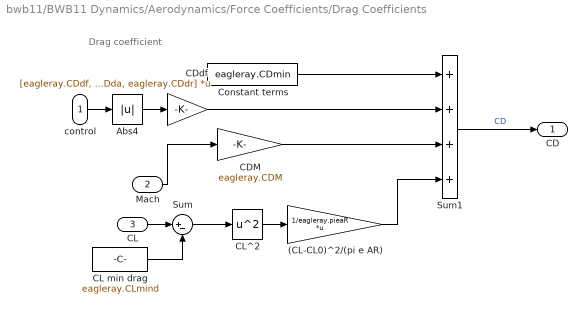
== system bwb11/BWB11 Dynamics/Aerodynamics/Force Coefficients/Drag Coefficients ==
  note: Drag coefficient
  control : Inport
  Mach : Inport  Port=2
  CL : Inport  Port=3  PortDimensions=1
  (CL-CL0)^2/(pi e AR) : Gain  Gain=1/eagleray.pieaR  Multiplication=Matrix(K*u)  SaturateOnIntegerOverflow=on  OutDataTypeStr=Inherit: Same as input  ParamDataTypeStr=Inherit: Same as input
  Abs4 : Abs  SaturateOnIntegerOverflow=on
  CDM : Gain  Gain=eagleray.CDM  SaturateOnIntegerOverflow=on  OutDataTypeStr=Inherit: Same as input  ParamDataTypeStr=Inherit: Same as input
  CDdf : Gain  Gain=[eagleray.CDdf, eagleray.CDde, eagleray.CDda, eagleray.CDdr]  Multiplication=Matrix(K*u)  SaturateOnIntegerOverflow=on  OutDataTypeStr=Inherit: Same as input  ParamDataTypeStr=Inherit: Same as input
  CL min drag : Constant  Value=eagleray.CLmind  VectorParams1D=off
  CL^2 : Math  Operator=square  SaturateOnIntegerOverflow=on
  Constant terms : Constant  Value=eagleray.CDmin  VectorParams1D=off
  Sum : Sum  Inputs=|+-  SaturateOnIntegerOverflow=on  InputSameDT=on  OutDataTypeStr=Inherit: Same as first input
  Sum1 : Sum  Inputs=++++  SaturateOnIntegerOverflow=on  InputSameDT=on  OutDataTypeStr=Inherit: Same as first input
  CD : Outport
  wires:
  (CL-CL0)^2/(pi e AR)/1 -> Sum1/4
  CL min drag/1 -> Sum/2
  CL/1 -> Sum/1
  Sum/1 -> CL^2/1
  CL^2/1 -> (CL-CL0)^2/(pi e AR)/1
  Sum1/1 -> CD/1  "CD"
  Mach/1 -> CDM/1
  control/1 -> Abs4/1
  Abs4/1 -> CDdf/1
  CDM/1 -> Sum1/3
  CDdf/1 -> Sum1/2
  Constant terms/1 -> Sum1/1

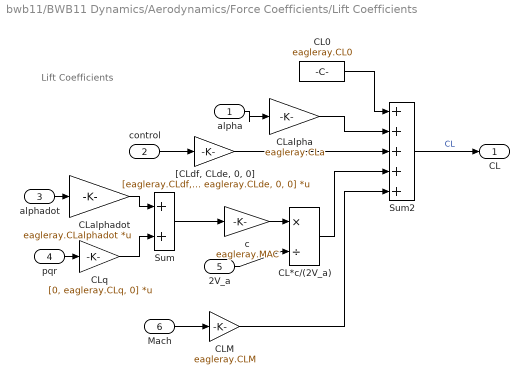
== system bwb11/BWB11 Dynamics/Aerodynamics/Force Coefficients/Lift Coefficients ==
  note: Lift Coefficients
  alpha : Inport
  control : Inport  Port=2
  alphadot : Inport  Port=3
  pqr : Inport  Port=4
  2V_a : Inport  Port=5
  Mach : Inport  Port=6
  CL*c/(2V_a) : Product  Inputs=*/  SaturateOnIntegerOverflow=on  InputSameDT=on  OutDataTypeStr=Inherit: Same as first input
  CL0 : Constant  Value=eagleray.CL0
  CLM : Gain  Gain=eagleray.CLM  SaturateOnIntegerOverflow=on  OutDataTypeStr=Inherit: Same as input  ParamDataTypeStr=Inherit: Same as input
  CLalpha : Gain  Gain=eagleray.CLa  SaturateOnIntegerOverflow=on  OutDataTypeStr=Inherit: Same as input  ParamDataTypeStr=Inherit: Same as input
  CLalphadot : Gain  Gain=eagleray.CLalphadot  Multiplication=Matrix(K*u)  SaturateOnIntegerOverflow=on  OutDataTypeStr=Inherit: Same as input  ParamDataTypeStr=Inherit: Same as input
  CLq : Gain  Gain=[0, eagleray.CLq, 0]  Multiplication=Matrix(K*u)  SaturateOnIntegerOverflow=on  OutDataTypeStr=Inherit: Same as input  ParamDataTypeStr=Inherit: Same as input
  Sum : Sum  SaturateOnIntegerOverflow=on  InputSameDT=on  OutDataTypeStr=Inherit: Same as first input
  Sum2 : Sum  Inputs=+++++  SaturateOnIntegerOverflow=on  InputSameDT=on  OutDataTypeStr=Inherit: Same as first input
  "[CLdf, CLde, 0, 0]" : Gain  Gain=[eagleray.CLdf, eagleray.CLde, 0, 0]  Multiplication=Matrix(K*u)  SaturateOnIntegerOverflow=on  OutDataTypeStr=Inherit: Same as input  ParamDataTypeStr=Inherit: Same as input
  c : Gain  Gain=eagleray.MAC  SaturateOnIntegerOverflow=on  OutDataTypeStr=Inherit: Same as input  ParamDataTypeStr=Inherit: Same as input
  CL : Outport
  wires:
  alphadot/1 -> CLalphadot/1
  alpha/1 -> CLalpha/1
  Mach/1 -> CLM/1
  2V_a/1 -> CL*c/(2V_a)/2
  pqr/1 -> CLq/1
  control/1 -> "[CLdf, CLde, 0, 0]"/1
  c/1 -> CL*c/(2V_a)/1
  CL*c/(2V_a)/1 -> Sum2/4
  CLM/1 -> Sum2/5
  Sum2/1 -> CL/1  "CL"
  "[CLdf, CLde, 0, 0]"/1 -> Sum2/3
  CLalpha/1 -> Sum2/2
  CL0/1 -> Sum2/1
  Sum/1 -> c/1
  CLalphadot/1 -> Sum/1
  CLq/1 -> Sum/2

== system bwb11/BWB11 Dynamics/Aerodynamics/Force Coefficients/Side Force Coefficients ==
  note: Side force coefficients
  beta : Inport
  control : Inport  Port=2
  angular rates : Inport  Port=3
  2V_a : Inport  Port=4
  CY*b/(2V_a) : Product  Inputs=*/  SaturateOnIntegerOverflow=on  InputSameDT=on  OutDataTypeStr=Inherit: Same as first input
  CYbeta : Gain  Gain=eagleray.CYbeta  SaturateOnIntegerOverflow=on  OutDataTypeStr=Inherit: Same as input  ParamDataTypeStr=Inherit: Same as input
  Sum3 : Sum  Inputs=+++  SaturateOnIntegerOverflow=on  InputSameDT=on  OutDataTypeStr=Inherit: Same as first input
  Wing span : Gain  Gain=eagleray.b  SaturateOnIntegerOverflow=on  OutDataTypeStr=Inherit: Same as input  ParamDataTypeStr=Inherit: Same as input
  "[0, 0, CYda, CYdr]" : Gain  Gain=[0, 0, eagleray.CYda, eagleray.CYdr]  Multiplication=Matrix(K*u)  SaturateOnIntegerOverflow=on  OutDataTypeStr=Inherit: Same as input  ParamDataTypeStr=Inherit: Same as input
  "[CYp, 0, CYr]" : Gain  Gain=[eagleray.CYp, 0,eagleray.CYr]  Multiplication=Matrix(K*u)  SaturateOnIntegerOverflow=on  OutDataTypeStr=Inherit: Same as input  ParamDataTypeStr=Inherit: Same as input
  CY : Outport
  wires:
  beta/1 -> CYbeta/1
  2V_a/1 -> CY*b/(2V_a)/2
  angular rates/1 -> "[CYp, 0, CYr]"/1
  control/1 -> "[0, 0, CYda, CYdr]"/1
  Wing span/1 -> CY*b/(2V_a)/1
  Sum3/1 -> CY/1  "CY"
  CY*b/(2V_a)/1 -> Sum3/3
  "[0, 0, CYda, CYdr]"/1 -> Sum3/2
  CYbeta/1 -> Sum3/1
  "[CYp, 0, CYr]"/1 -> Wing span/1

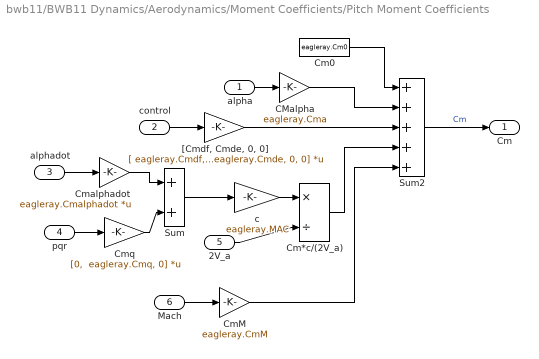
== system bwb11/BWB11 Dynamics/Aerodynamics/Moment Coefficients/Pitch Moment Coefficients ==
  alpha : Inport
  control : Inport  Port=2
  alphadot : Inport  Port=3
  pqr : Inport  Port=4
  2V_a : Inport  Port=5
  Mach : Inport  Port=6
  CMalpha : Gain  Gain=eagleray.Cma  SaturateOnIntegerOverflow=on  OutDataTypeStr=Inherit: Same as input  ParamDataTypeStr=Inherit: Same as input
  Cm*c/(2V_a) : Product  Inputs=*/  SaturateOnIntegerOverflow=on  InputSameDT=on  OutDataTypeStr=Inherit: Same as first input
  Cm0 : Constant  Value=eagleray.Cm0
  CmM : Gain  Gain=eagleray.CmM  SaturateOnIntegerOverflow=on  OutDataTypeStr=Inherit: Same as input  ParamDataTypeStr=Inherit: Same as input
  Cmalphadot : Gain  Gain=eagleray.Cmalphadot  Multiplication=Matrix(K*u)  SaturateOnIntegerOverflow=on  OutDataTypeStr=Inherit: Same as input  ParamDataTypeStr=Inherit: Same as input
  Cmq : Gain  Gain="[0,  eagleray.Cmq, 0]"  Multiplication=Matrix(K*u)  SaturateOnIntegerOverflow=on  OutDataTypeStr=Inherit: Same as input  ParamDataTypeStr=Inherit: Same as input
  Sum : Sum  SaturateOnIntegerOverflow=on  InputSameDT=on  OutDataTypeStr=Inherit: Same as first input
  Sum2 : Sum  Inputs=+++++  SaturateOnIntegerOverflow=on  InputSameDT=on  OutDataTypeStr=Inherit: Same as first input
  "[Cmdf, Cmde, 0, 0]" : Gain  Gain="[ eagleray.Cmdf,  eagleray.Cmde, 0, 0]"  Multiplication=Matrix(K*u)  SaturateOnIntegerOverflow=on  OutDataTypeStr=Inherit: Same as input  ParamDataTypeStr=Inherit: Same as input
  c : Gain  Gain=eagleray.MAC  SaturateOnIntegerOverflow=on  OutDataTypeStr=Inherit: Same as input  ParamDataTypeStr=Inherit: Same as input
  Cm : Outport
  wires:
  Cmq/1 -> Sum/2
  Cmalphadot/1 -> Sum/1
  Sum/1 -> c/1
  Cm0/1 -> Sum2/1
  CMalpha/1 -> Sum2/2
  "[Cmdf, Cmde, 0, 0]"/1 -> Sum2/3
  Sum2/1 -> Cm/1  "Cm"
  CmM/1 -> Sum2/5
  Cm*c/(2V_a)/1 -> Sum2/4
  c/1 -> Cm*c/(2V_a)/1
  control/1 -> "[Cmdf, Cmde, 0, 0]"/1
  pqr/1 -> Cmq/1
  2V_a/1 -> Cm*c/(2V_a)/2
  Mach/1 -> CmM/1
  alpha/1 -> CMalpha/1
  alphadot/1 -> Cmalphadot/1

== system bwb11/BWB11 Dynamics/Aerodynamics/Moment Coefficients/Roll Moment Coefficients ==
  note: Roll moment coefficient
  beta : Inport
  control : Inport  Port=2
  angular rates : Inport  Port=3
  2V : Inport  Port=4
  CY*b/(2V) : Product  Inputs=*/  SaturateOnIntegerOverflow=on  InputSameDT=on  OutDataTypeStr=Inherit: Same as first input
  Clbeta : Gain  Gain=eagleray.Clbeta  SaturateOnIntegerOverflow=on  OutDataTypeStr=Inherit: Same as input  ParamDataTypeStr=Inherit: Same as input
  Sum3 : Sum  Inputs=+++  SaturateOnIntegerOverflow=on  InputSameDT=on  OutDataTypeStr=Inherit: Same as first input
  Wing span : Gain  Gain=eagleray.b  SaturateOnIntegerOverflow=on  OutDataTypeStr=Inherit: Same as input  ParamDataTypeStr=Inherit: Same as input
  "[0, 0, Clda, Cldr]" : Gain  Gain="[0, 0,  eagleray.Clda,  eagleray.Cldr]"  Multiplication=Matrix(K*u)  SaturateOnIntegerOverflow=on  OutDataTypeStr=Inherit: Same as input  ParamDataTypeStr=Inherit: Same as input
  "[Clp, 0, Clr]" : Gain  Gain="[ eagleray.Clp, 0,  eagleray.Clr]"  Multiplication=Matrix(K*u)  SaturateOnIntegerOverflow=on  OutDataTypeStr=Inherit: Same as input  ParamDataTypeStr=Inherit: Same as input
  Cl : Outport
  wires:
  "[Clp, 0, Clr]"/1 -> Wing span/1
  Clbeta/1 -> Sum3/1
  "[0, 0, Clda, Cldr]"/1 -> Sum3/2
  CY*b/(2V)/1 -> Sum3/3
  Sum3/1 -> Cl/1  "Cl"
  Wing span/1 -> CY*b/(2V)/1
  control/1 -> "[0, 0, Clda, Cldr]"/1
  angular rates/1 -> "[Clp, 0, Clr]"/1
  2V/1 -> CY*b/(2V)/2
  beta/1 -> Clbeta/1

== system bwb11/BWB11 Dynamics/Aerodynamics/Moment Coefficients/Yaw Moment Coefficients ==
  note: Yaw moment coefficient
  beta : Inport
  control : Inport  Port=2
  angular rates : Inport  Port=3
  2V_a : Inport  Port=4
  Cn*b/(2V_a) : Product  Inputs=*/  SaturateOnIntegerOverflow=on  InputSameDT=on  OutDataTypeStr=Inherit: Same as first input
  Cnbeta : Gain  Gain=eagleray.Cnbeta  SaturateOnIntegerOverflow=on  OutDataTypeStr=Inherit: Same as input  ParamDataTypeStr=Inherit: Same as input
  Sum3 : Sum  Inputs=+++  SaturateOnIntegerOverflow=on  InputSameDT=on  OutDataTypeStr=Inherit: Same as first input
  Wing span : Gain  Gain=eagleray.b  SaturateOnIntegerOverflow=on  OutDataTypeStr=Inherit: Same as input  ParamDataTypeStr=Inherit: Same as input
  "[0, 0, Cnda, Cndr]" : Gain  Gain="[0, 0,  eagleray.Cnda,  eagleray.Cndr]"  Multiplication=Matrix(K*u)  SaturateOnIntegerOverflow=on  OutDataTypeStr=Inherit: Same as input  ParamDataTypeStr=Inherit: Same as input
  "[Cnp, 0, Cnr]" : Gain  Gain="[ eagleray.Cnp, 0,  eagleray.Cnr]"  Multiplication=Matrix(K*u)  SaturateOnIntegerOverflow=on  OutDataTypeStr=Inherit: Same as input  ParamDataTypeStr=Inherit: Same as input
  Cn : Outport
  wires:
  beta/1 -> Cnbeta/1
  2V_a/1 -> Cn*b/(2V_a)/2
  angular rates/1 -> "[Cnp, 0, Cnr]"/1
  control/1 -> "[0, 0, Cnda, Cndr]"/1
  Wing span/1 -> Cn*b/(2V_a)/1
  Sum3/1 -> Cn/1  "Cn"
  Cn*b/(2V_a)/1 -> Sum3/3
  "[0, 0, Cnda, Cndr]"/1 -> Sum3/2
  Cnbeta/1 -> Sum3/1
  "[Cnp, 0, Cnr]"/1 -> Wing span/1

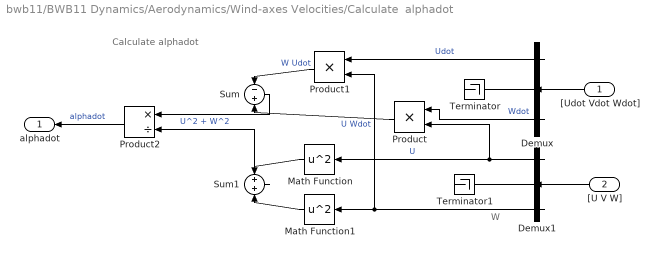
== system bwb11/BWB11 Dynamics/Aerodynamics/Wind-axes Velocities/Calculate  alphadot ==
  note: Calculate alphadot
  note: W
  "[Udot Vdot Wdot]" : Inport
  "[U V W]" : Inport  Port=2
  Demux : Demux  Outputs=3
  Demux1 : Demux  Outputs=3
  Math Function : Math  Operator=square  SaturateOnIntegerOverflow=on
  Math Function1 : Math  Operator=square  SaturateOnIntegerOverflow=on
  Product : Product  RndMeth=Zero
  Product1 : Product  RndMeth=Zero
  Product2 : Product  Inputs=*/  RndMeth=Zero
  Sum : Sum  Inputs=-|+
  Sum1 : Sum  Inputs=+|+
  Terminator : Terminator
  Terminator1 : Terminator
  alphadot : Outport
  wires:
  Product2/1 -> alphadot/1  "alphadot"
  "[Udot Vdot Wdot]"/1 -> Demux/1
  "[U V W]"/1 -> Demux1/1
  Demux1/2 -> Terminator1/1
  Sum/1 -> Product2/1
  Product/1 -> Sum/2  "U Wdot"
  Product1/1 -> Sum/1  "W Udot"
  Sum1/1 -> Product2/2  "U^2 + W^2"
  Math Function1/1 -> Sum1/2
  Math Function/1 -> Sum1/1
  Demux1/3 -> Math Function1/1, Product1/2
  Demux1/1 -> Math Function/1, Product/2  "U"
  Demux/2 -> Terminator/1
  Demux/3 -> Product/1  "Wdot"
  Demux/1 -> Product1/1  "Udot"

== system bwb11/BWB11 Dynamics/Forces and moments/Aerodynamic Forces and Moments/3x3 Cross Product ==
  A : Inport
  B : Inport  Port=2
  "A " : InportShadow  Port=1
  "B " : InportShadow  Port=2
  Subsystem : Subsystem
  Subsystem1 : Subsystem
  Sum : Sum  Inputs=+|-  SaturateOnIntegerOverflow=on  InputSameDT=on  OutDataTypeStr=Inherit: Same as first input
  C : Outport
  wires:
  "B "/1 -> Subsystem1/2(B)
  "A "/1 -> Subsystem1/1(A)
  Sum/1 -> C/1
  B/1 -> Subsystem/2(B)
  A/1 -> Subsystem/1(A)
  Subsystem/1(Out1) -> Sum/1
  Subsystem1/1(Out1) -> Sum/2

== system bwb11/BWB11 Dynamics/Forces and moments/Total Moment/Moments about CG  due to Propulsion   Forces ==
  Forces : Inport
  CG : Inport  Port=2
  3x3 Cross Product : aerolibutil/3x3 Cross Product
  Sum : Sum  Inputs=|+-  SaturateOnIntegerOverflow=on
  constant : Constant  Value=0
  Moments : Outport
  wires:
  Sum/1 -> 3x3 Cross Product/2
  Forces/1 -> 3x3 Cross Product/1
  3x3 Cross Product/1 -> Moments/1
  CG/1 -> Sum/1
  constant/1 -> Sum/2

== system bwb11/BWB11 Dynamics/Forces and moments/Aerodynamic Forces and Moments/3x3 Cross Product/Subsystem ==
  A : Inport
  B : Inport  Port=2
  Demux : Demux  Outputs=3
  Demux1 : Demux  Outputs=3
  Mux : Mux  Inputs=3
  i x j : Product  SaturateOnIntegerOverflow=on  InputSameDT=on  OutDataTypeStr=Inherit: Same as first input
  j x k : Product  SaturateOnIntegerOverflow=on  InputSameDT=on  OutDataTypeStr=Inherit: Same as first input
  k x i : Product  SaturateOnIntegerOverflow=on  InputSameDT=on  OutDataTypeStr=Inherit: Same as first input
  Out1 : Outport
  wires:
  Demux1/3 -> j x k/2
  Demux/2 -> j x k/1
  Demux/3 -> k x i/1
  Demux1/1 -> k x i/2
  Demux1/2 -> i x j/2
  Demux/1 -> i x j/1
  i x j/1 -> Mux/3
  k x i/1 -> Mux/2
  j x k/1 -> Mux/1
  B/1 -> Demux1/1
  A/1 -> Demux/1
  Mux/1 -> Out1/1

== system bwb11/BWB11 Dynamics/Forces and moments/Aerodynamic Forces and Moments/3x3 Cross Product/Subsystem1 ==
  A : Inport
  B : Inport  Port=2
  Demux : Demux  Outputs=3
  Demux1 : Demux  Outputs=3
  Mux : Mux  Inputs=3
  i x k : Product  SaturateOnIntegerOverflow=on  InputSameDT=on  OutDataTypeStr=Inherit: Same as first input
  j x i : Product  SaturateOnIntegerOverflow=on  InputSameDT=on  OutDataTypeStr=Inherit: Same as first input
  k x j : Product  SaturateOnIntegerOverflow=on  InputSameDT=on  OutDataTypeStr=Inherit: Same as first input
  Out1 : Outport
  wires:
  j x i/1 -> Mux/3
  i x k/1 -> Mux/2
  k x j/1 -> Mux/1
  Mux/1 -> Out1/1
  Demux1/1 -> j x i/2
  Demux/2 -> j x i/1
  Demux1/3 -> i x k/2
  Demux/1 -> i x k/1
  Demux1/2 -> k x j/2
  Demux/3 -> k x j/1
  B/1 -> Demux1/1
  A/1 -> Demux/1
